simulink subsystem "Final_Project_PreAlign_20260605_152612"  (R2024a)
settings: Solver=VariableStepAuto  StartTime=0.0  StopTime=10.0  RelTol=1e-3
values from neighbouring files (symbols this model uses):
  D = hypot(Ep(:,1)-Tp(:,1)',Ep(:,2)-Tp(:,2)')    [pp_compare_stage.m]    (also in pp_diag_path.m; pp_t09_clear.m = hypot(Ep(:,1)-Tperim(:,1)', Ep(:,2)-Tperim(:,2)'); pp_tune2.m)
undefined symbols (not defined in the file or in its folder): waypoint_const
libraries: CarMaker4SL x83, simulink x2
(part 2 of 5)

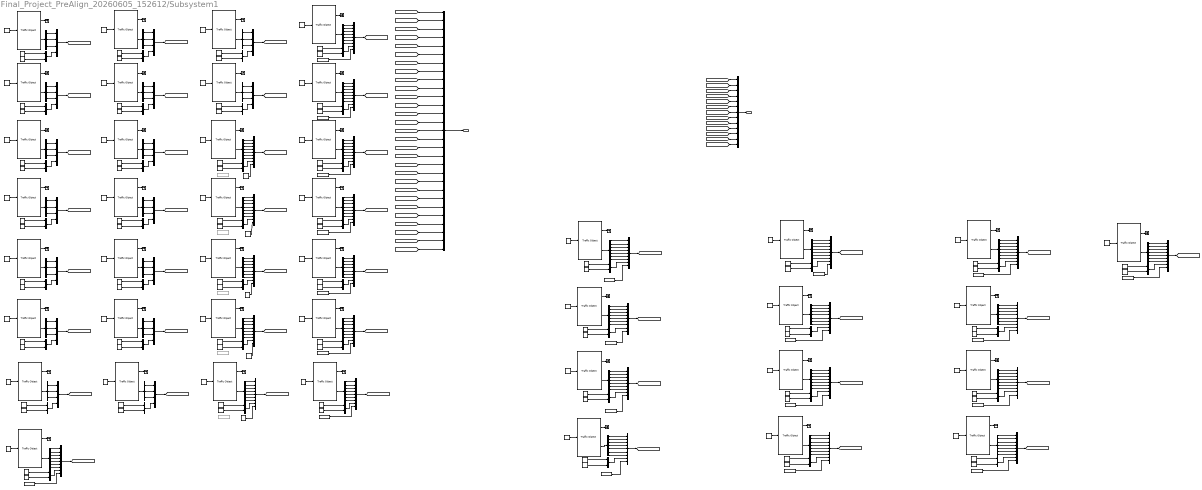
== system Final_Project_PreAlign_20260605_152612/Subsystem1 ==
  Bus Creator{,1,3..13} (13 alike) : BusCreator  Inputs=9  OutDataTypeStr=Bus: TrafficObjBus
  Bus Creator2 : BusCreator  Inputs=13  OutDataTypeStr=Bus: AllTrafficBus
  Bus Selector{,1..5,10..13,16..17,20..21,24..25} (16 alike) : BusSelector  OutputSignals=t_0 x,t_0 y,r_zyx z
  Bus Selector{6..9,14..15,18..19,22..23,26..41} (26 alike) : BusSelector  OutputSignals=t_0 x,t_0 y,r_zyx z,v_0 x,v_0 y,a_0 x,a_0 y
  Constant1 : Constant  Value=8
  Constant10 : Constant  Value=7
  Constant100 : Constant  Value=21
  Constant{7,9,12,14,16,18,20,22,30..31,34,38,42,44,47..48,51,53,59..60,63,65,71..72,75,77,83..85,89..90,95..96,101,103,108..109,113..114,119..120,125} (42 alike) : Constant  Value=4.47
  Constant102 : Constant  Value=16
  Constant{5,8,11,13,15,17,19,21,23,28,33,35,37,39,43,45,50,52,54,57,62,64,66,69,74,76,78,81,86,91..92,97..98,104..105,110..111,115..116,121..122,126} (42 alike) : Constant  Value=1.97
  Constant106 : Constant  Value=22
  Constant107 : Constant  Value=23
  Constant112 : Constant  Value=25
  Constant117 : Constant  Value=26
  Constant118 : Constant  Value=27
  Constant123 : Constant  Value=24
  Constant124 : Constant  Value=28
  Constant{36,131..135} (6 alike) : Constant  Value=0
  Constant2 : Constant  Value=9
  Constant24 : Constant  Value=22
  Constant25 : Constant  Value=23
  Constant26 : Constant  Value=2
  Constant27 : Constant
  Constant29 : Constant  Value=16
  Constant3 : Constant  Value=14
  Constant32 : Constant  Value=10
  Constant4 : Constant  Value=15
  Constant40 : Constant  Value=24
  Constant41 : Constant  Value=3
  Constant46 : Constant  Value=17
  Constant49 : Constant  Value=11
  Constant55 : Constant  Value=25
  Constant56 : Constant  Value=4
  Constant58 : Constant  Value=18
  Constant6 : Constant  Value=21
  Constant61 : Constant  Value=12
  Constant67 : Constant  Value=26
  Constant68 : Constant  Value=5
  Constant70 : Constant  Value=19
  Constant73 : Constant  Value=13
  Constant79 : Constant  Value=27
  Constant80 : Constant  Value=6
  Constant82 : Constant  Value=20
  Constant87 : Constant  Value=28
  Constant88 : Constant  Value=17
  Constant93 : Constant  Value=18
  Constant94 : Constant  Value=19
  Constant99 : Constant  Value=20
  Mux{1,4,6,8,11,14,16,18..19,21,23,26,28,30,32..33,35,38..39,41,43,46..47,49,51,54..55,57..58,60..72} (42 alike) : Mux  Inputs=2
  Mux{2..3,5,7,10,13,22,25,27,29,34,37,42,45,50,53} (16 alike) : Mux
  Mux{12,15,17,20,24,31,36,40,44,48,52,56,59} (13 alike) : Mux  Inputs=9
  Mux9 : Mux  Inputs=29
  Read CM Dict : CarMaker4SL/Read CM Dict  xname=Traffic.T27.rzv  xsync=off  xstime=Continuous
  Read CM Dict1 : CarMaker4SL/Read CM Dict  Commented=on  xname=Traffic.T16.rzv  xsync=off  xstime=Continuous
  Read CM Dict10 : CarMaker4SL/Read CM Dict  xname=Traffic.T25.rzv  xsync=off  xstime=Continuous
  Read CM Dict11 : CarMaker4SL/Read CM Dict  xname=Traffic.T26.rzv  xsync=off  xstime=Continuous
  Read CM Dict12 : CarMaker4SL/Read CM Dict  xname=Traffic.T28.rzv  xsync=off  xstime=Continuous
  Read CM Dict13 : CarMaker4SL/Read CM Dict  xname=Traffic.T17.rzv  xsync=off  xstime=Continuous
  Read CM Dict14 : CarMaker4SL/Read CM Dict  xname=Traffic.T19.rzv  xsync=off  xstime=Continuous
  Read CM Dict15 : CarMaker4SL/Read CM Dict  xname=Traffic.T18.rzv  xsync=off  xstime=Continuous
  Read CM Dict16 : CarMaker4SL/Read CM Dict  xname=Traffic.T16.rzv  xsync=off  xstime=Continuous
  Read CM Dict17 : CarMaker4SL/Read CM Dict  xname=Traffic.T21.rzv  xsync=off  xstime=Continuous
  Read CM Dict18 : CarMaker4SL/Read CM Dict  xname=Traffic.T23.rzv  xsync=off  xstime=Continuous
  Read CM Dict19 : CarMaker4SL/Read CM Dict  xname=Traffic.T22.rzv  xsync=off  xstime=Continuous
  Read CM Dict2 : CarMaker4SL/Read CM Dict  Commented=on  xname=Traffic.T17.rzv  xsync=off  xstime=Continuous
  Read CM Dict20 : CarMaker4SL/Read CM Dict  xname=Traffic.T20.rzv  xsync=off  xstime=Continuous
  Read CM Dict21 : CarMaker4SL/Read CM Dict  xname=Traffic.T25.rzv  xsync=off  xstime=Continuous
  Read CM Dict22 : CarMaker4SL/Read CM Dict  xname=Traffic.T27.rzv  xsync=off  xstime=Continuous
  Read CM Dict23 : CarMaker4SL/Read CM Dict  xname=Traffic.T26.rzv  xsync=off  xstime=Continuous
  Read CM Dict24 : CarMaker4SL/Read CM Dict  xname=Traffic.T24.rzv  xsync=off  xstime=Continuous
  Read CM Dict25 : CarMaker4SL/Read CM Dict  xname=Traffic.T28.rzv  xsync=off  xstime=Continuous
  Read CM Dict3 : CarMaker4SL/Read CM Dict  Commented=on  xname=Traffic.T18.rzv  xsync=off  xstime=Continuous
  Read CM Dict4 : CarMaker4SL/Read CM Dict  Commented=on  xname=Traffic.T19.rzv  xsync=off  xstime=Continuous
  Read CM Dict5 : CarMaker4SL/Read CM Dict  Commented=on  xname=Traffic.T20.rzv  xsync=off  xstime=Continuous
  Read CM Dict6 : CarMaker4SL/Read CM Dict  xname=Traffic.T21.rzv  xsync=off  xstime=Continuous
  Read CM Dict7 : CarMaker4SL/Read CM Dict  xname=Traffic.T22.rzv  xsync=off  xstime=Continuous
  Read CM Dict8 : CarMaker4SL/Read CM Dict  xname=Traffic.T23.rzv  xsync=off  xstime=Continuous
  Read CM Dict9 : CarMaker4SL/Read CM Dict  xname=Traffic.T24.rzv  xsync=off  xstime=Continuous
  Terminator{1..42} (42 alike) : Terminator
  Traffic Object1 : CarMaker4SL/Traffic Object  xname=T07  ximode=Traffic Id  xstime=Inherited
      settings: SourceProductName=CarMaker4SL
  Traffic Object10 : CarMaker4SL/Traffic Object  xname=T23  ximode=Traffic Id  xstime=Inherited
      settings: SourceProductName=CarMaker4SL
  Traffic Object11 : CarMaker4SL/Traffic Object  xname=T03  ximode=Traffic Id  xstime=Inherited
      settings: SourceProductName=CarMaker4SL
  Traffic Object12 : CarMaker4SL/Traffic Object  xname=T10  ximode=Traffic Id  xstime=Inherited
      settings: SourceProductName=CarMaker4SL
  Traffic Object13 : CarMaker4SL/Traffic Object  xname=T00  ximode=Traffic Id  xstime=Inherited
      settings: SourceProductName=CarMaker4SL
  Traffic Object14 : CarMaker4SL/Traffic Object  xname=T17  ximode=Traffic Id  xstime=Inherited
      settings: SourceProductName=CarMaker4SL
  Traffic Object15 : CarMaker4SL/Traffic Object  xname=T01  ximode=Traffic Id  xstime=Inherited
      settings: SourceProductName=CarMaker4SL
  Traffic Object16 : CarMaker4SL/Traffic Object  xname=T24  ximode=Traffic Id  xstime=Inherited
      settings: SourceProductName=CarMaker4SL
  Traffic Object17 : CarMaker4SL/Traffic Object  xname=T04  ximode=Traffic Id  xstime=Inherited
      settings: SourceProductName=CarMaker4SL
  Traffic Object18 : CarMaker4SL/Traffic Object  xname=T11  ximode=Traffic Id  xstime=Inherited
      settings: SourceProductName=CarMaker4SL
  Traffic Object19 : CarMaker4SL/Traffic Object  xname=T18  ximode=Traffic Id  xstime=Inherited
      settings: SourceProductName=CarMaker4SL
  Traffic Object2 : CarMaker4SL/Traffic Object  xname=T08  ximode=Traffic Id  xstime=Inherited
      settings: SourceProductName=CarMaker4SL
  Traffic Object20 : CarMaker4SL/Traffic Object  xname=T25  ximode=Traffic Id  xstime=Inherited
      settings: SourceProductName=CarMaker4SL
  Traffic Object21 : CarMaker4SL/Traffic Object  xname=T05  ximode=Traffic Id  xstime=Inherited
      settings: SourceProductName=CarMaker4SL
  Traffic Object22 : CarMaker4SL/Traffic Object  xname=T12  ximode=Traffic Id  xstime=Inherited
      settings: SourceProductName=CarMaker4SL
  Traffic Object23 : CarMaker4SL/Traffic Object  xname=T19  ximode=Traffic Id  xstime=Inherited
      settings: SourceProductName=CarMaker4SL
  Traffic Object24 : CarMaker4SL/Traffic Object  xname=T26  ximode=Traffic Id  xstime=Inherited
      settings: SourceProductName=CarMaker4SL
  Traffic Object25 : CarMaker4SL/Traffic Object  xname=T06  ximode=Traffic Id  xstime=Inherited
      settings: SourceProductName=CarMaker4SL
  Traffic Object26 : CarMaker4SL/Traffic Object  xname=T13  ximode=Traffic Id  xstime=Inherited
      settings: SourceProductName=CarMaker4SL
  Traffic Object27 : CarMaker4SL/Traffic Object  xname=T20  ximode=Traffic Id  xstime=Inherited
      settings: SourceProductName=CarMaker4SL
  Traffic Object28 : CarMaker4SL/Traffic Object  xname=T27  ximode=Traffic Id  xstime=Inherited
      settings: SourceProductName=CarMaker4SL
  Traffic Object29 : CarMaker4SL/Traffic Object  xname=T28  ximode=Traffic Id  xstime=Inherited
      settings: SourceProductName=CarMaker4SL
  Traffic Object3 : CarMaker4SL/Traffic Object  xname=T02  ximode=Traffic Id  xstime=Inherited
      settings: SourceProductName=CarMaker4SL
  Traffic Object30 : CarMaker4SL/Traffic Object  xname=T17  ximode=Traffic Id  xstime=Inherited
      settings: SourceProductName=CarMaker4SL
  Traffic Object31 : CarMaker4SL/Traffic Object  xname=T19  ximode=Traffic Id  xstime=Inherited
      settings: SourceProductName=CarMaker4SL
  Traffic Object32 : CarMaker4SL/Traffic Object  xname=T18  ximode=Traffic Id  xstime=Inherited
      settings: SourceProductName=CarMaker4SL
  Traffic Object33 : CarMaker4SL/Traffic Object  xname=T21  ximode=Traffic Id  xstime=Inherited
      settings: SourceProductName=CarMaker4SL
  Traffic Object34 : CarMaker4SL/Traffic Object  xname=T23  ximode=Traffic Id  xstime=Inherited
      settings: SourceProductName=CarMaker4SL
  Traffic Object35 : CarMaker4SL/Traffic Object  xname=T16  ximode=Traffic Id  xstime=Inherited
      settings: SourceProductName=CarMaker4SL
  Traffic Object36 : CarMaker4SL/Traffic Object  xname=T22  ximode=Traffic Id  xstime=Inherited
      settings: SourceProductName=CarMaker4SL
  Traffic Object37 : CarMaker4SL/Traffic Object  xname=T20  ximode=Traffic Id  xstime=Inherited
      settings: SourceProductName=CarMaker4SL
  Traffic Object38 : CarMaker4SL/Traffic Object  xname=T25  ximode=Traffic Id  xstime=Inherited
      settings: SourceProductName=CarMaker4SL
  Traffic Object39 : CarMaker4SL/Traffic Object  xname=T27  ximode=Traffic Id  xstime=Inherited
      settings: SourceProductName=CarMaker4SL
  Traffic Object4 : CarMaker4SL/Traffic Object  xname=T14  ximode=Traffic Id  xstime=Inherited
      settings: SourceProductName=CarMaker4SL
  Traffic Object40 : CarMaker4SL/Traffic Object  xname=T26  ximode=Traffic Id  xstime=Inherited
      settings: SourceProductName=CarMaker4SL
  Traffic Object41 : CarMaker4SL/Traffic Object  xname=T24  ximode=Traffic Id  xstime=Inherited
      settings: SourceProductName=CarMaker4SL
  Traffic Object42 : CarMaker4SL/Traffic Object  xname=T28  ximode=Traffic Id  xstime=Inherited
      settings: SourceProductName=CarMaker4SL
  Traffic Object5 : CarMaker4SL/Traffic Object  xname=T15  ximode=Traffic Id  xstime=Inherited
      settings: SourceProductName=CarMaker4SL
  Traffic Object6 : CarMaker4SL/Traffic Object  xname=T09  ximode=Traffic Id  xstime=Inherited
      settings: SourceProductName=CarMaker4SL
  Traffic Object7 : CarMaker4SL/Traffic Object  xname=T21  ximode=Traffic Id  xstime=Inherited
      settings: SourceProductName=CarMaker4SL
  Traffic Object8 : CarMaker4SL/Traffic Object  xname=T22  ximode=Traffic Id  xstime=Inherited
      settings: SourceProductName=CarMaker4SL
  Traffic Object9 : CarMaker4SL/Traffic Object  xname=T16  ximode=Traffic Id  xstime=Inherited
      settings: SourceProductName=CarMaker4SL
  Traffic_Info : Outport
  Outport : Outport  Port=2
  wires:
  Constant135/1 -> Mux56/9
  Constant134/1 -> Mux48/9
  Constant133/1 -> Mux40/9
  Constant132/1 -> Mux31/9
  Constant131/1 -> Mux20/9
  Read CM Dict16/1 -> Bus Creator/9
  Read CM Dict13/1 -> Bus Creator3/9
  Read CM Dict15/1 -> Bus Creator1/9
  Read CM Dict14/1 -> Bus Creator4/9
  Read CM Dict20/1 -> Bus Creator5/9
  [Traffic_Info_16_Bus] -> Bus Creator2/1  "t16"
  [Traffic_Info_17_Bus] -> Bus Creator2/2  "t17"
  [Traffic_Info_18_Bus] -> Bus Creator2/3  "t18"
  [Traffic_Info_19_Bus] -> Bus Creator2/4  "t19"
  [Traffic_Info_20_Bus] -> Bus Creator2/5  "t20"
  [Traffic_Info_21_Bus] -> Bus Creator2/6  "t21"
  [Traffic_Info_22_Bus] -> Bus Creator2/7  "t22"
  [Traffic_Info_23_Bus] -> Bus Creator2/8  "t23"
  [Traffic_Info_24_Bus] -> Bus Creator2/9  "t24"
  [Traffic_Info_25_Bus] -> Bus Creator2/10  "t25"
  [Traffic_Info_26_Bus] -> Bus Creator2/11  "t26"
  [Traffic_Info_27_Bus] -> Bus Creator2/12  "t27"
  [Traffic_Info_28_Bus] -> Bus Creator2/13  "t28"
  Bus Selector41/7 -> Bus Creator13/7  "<a_0 y>"
  Bus Selector41/1 -> Bus Creator13/1  "<t_0 x>"
  Constant125/1 -> Mux72/1
  Bus Selector41/2 -> Bus Creator13/2  "<t_0 y>"
  Traffic Object42/1 -> Terminator42/1
  Bus Selector41/6 -> Bus Creator13/6  "<a_0 x>"
  Traffic Object42/2 -> Bus Selector41/1
  Bus Creator13/1 -> [Traffic_Info_28_Bus]
  Mux72/1 -> Bus Creator13/8  "Traffic_Boundary"
  Bus Selector41/4 -> Bus Creator13/4  "<v_0 x>"
  Constant126/1 -> Mux72/2
  Bus Selector41/5 -> Bus Creator13/5  "<v_0 y>"
  Bus Selector41/3 -> Bus Creator13/3  "<r_zyx z>"
  Read CM Dict25/1 -> Bus Creator13/9  "Yawrate"
  Constant124/1 -> Traffic Object42/1
  Constant114/1 -> Mux70/1
  Bus Selector39/3 -> Bus Creator10/3  "<r_zyx z>"
  Constant116/1 -> Mux68/2
  Bus Creator12/1 -> [Traffic_Info_27_Bus]
  Mux71/1 -> Bus Creator10/8  "Traffic_Boundary"
  Bus Selector39/7 -> Bus Creator10/7  "<a_0 y>"
  Traffic Object39/1 -> Terminator39/1
  Traffic Object41/2 -> Bus Selector40/1
  Bus Selector38/2 -> Bus Creator12/2  "<t_0 y>"
  Mux68/1 -> Bus Creator11/8  "Traffic_Boundary"
  Bus Selector40/6 -> Bus Creator9/6  "<a_0 x>"
  Traffic Object39/2 -> Bus Selector38/1
  Bus Selector37/5 -> Bus Creator11/5  "<v_0 y>"
  Bus Selector37/7 -> Bus Creator11/7  "<a_0 y>"
  Bus Selector40/4 -> Bus Creator9/4  "<v_0 x>"
  Traffic Object38/2 -> Bus Selector37/1
  Bus Selector39/2 -> Bus Creator10/2  "<t_0 y>"
  Constant112/1 -> Traffic Object38/1
  Bus Selector40/3 -> Bus Creator9/3  "<r_zyx z>"
  Constant119/1 -> Mux69/1
  Bus Selector40/5 -> Bus Creator9/5  "<v_0 y>"
  Traffic Object40/2 -> Bus Selector39/1
  Bus Selector38/1 -> Bus Creator12/1  "<t_0 x>"
  Constant120/1 -> Mux71/1
  Bus Selector38/7 -> Bus Creator12/7  "<a_0 y>"
  Bus Selector40/2 -> Bus Creator9/2  "<t_0 y>"
  Traffic Object40/1 -> Terminator40/1
  Constant117/1 -> Traffic Object40/1
  Bus Selector40/1 -> Bus Creator9/1  "<t_0 x>"
  Read CM Dict23/1 -> Bus Creator10/9  "Yawrate"
  Constant115/1 -> Mux70/2
  Bus Selector39/1 -> Bus Creator10/1  "<t_0 x>"
  Bus Selector39/6 -> Bus Creator10/6  "<a_0 x>"
  Constant121/1 -> Mux71/2
  Constant118/1 -> Traffic Object39/1
  Bus Selector37/4 -> Bus Creator11/4  "<v_0 x>"
  Constant113/1 -> Mux68/1
  Read CM Dict24/1 -> Bus Creator9/9  "Yawrate"
  Bus Selector40/7 -> Bus Creator9/7  "<a_0 y>"
  Bus Selector37/3 -> Bus Creator11/3  "<r_zyx z>"
  Bus Selector39/5 -> Bus Creator10/5  "<v_0 y>"
  Read CM Dict22/1 -> Bus Creator12/9  "Yawrate"
  Bus Selector37/2 -> Bus Creator11/2  "<t_0 y>"
  Bus Creator11/1 -> [Traffic_Info_25_Bus]
  Read CM Dict21/1 -> Bus Creator11/9  "Yawrate"
  Mux70/1 -> Bus Creator9/8  "Traffic_Boundary"
  Bus Selector37/6 -> Bus Creator11/6  "<a_0 x>"
  Bus Selector38/3 -> Bus Creator12/3  "<r_zyx z>"
  Bus Selector37/1 -> Bus Creator11/1  "<t_0 x>"
  Bus Creator9/1 -> [Traffic_Info_24_Bus]
  Traffic Object38/1 -> Terminator38/1
  Constant122/1 -> Mux69/2
  Bus Selector38/6 -> Bus Creator12/6  "<a_0 x>"
  Bus Creator10/1 -> [Traffic_Info_26_Bus]
  Bus Selector38/4 -> Bus Creator12/4  "<v_0 x>"
  Bus Selector38/5 -> Bus Creator12/5  "<v_0 y>"
  Constant123/1 -> Traffic Object41/1
  Traffic Object41/1 -> Terminator41/1
  Bus Selector39/4 -> Bus Creator10/4  "<v_0 x>"
  Mux69/1 -> Bus Creator12/8  "Traffic_Boundary"
  Constant105/1 -> Mux64/2
  Mux65/1 -> Bus Creator8/8  "Traffic_Boundary"
  Bus Selector34/1 -> Bus Creator8/1  "<t_0 x>"
  Traffic Object36/2 -> Bus Selector35/1
  Read CM Dict19/1 -> Bus Creator6/9  "Yawrate"
  Bus Selector32/1 -> Bus Creator7/1  "<t_0 x>"
  Bus Creator6/1 -> [Traffic_Info_22_Bus]
  Bus Selector34/4 -> Bus Creator8/4  "<v_0 x>"
  Bus Creator8/1 -> [Traffic_Info_23_Bus]
  Bus Selector35/4 -> Bus Creator6/4  "<v_0 x>"
  Traffic Object37/1 -> Terminator37/1
  Constant111/1 -> Mux65/2
  Constant99/1 -> Traffic Object37/1
  Bus Selector34/6 -> Bus Creator8/6  "<a_0 x>"
  Bus Selector34/5 -> Bus Creator8/5  "<v_0 y>"
  Mux64/1 -> Bus Creator7/8  "Traffic_Boundary"
  Bus Creator7/1 -> [Traffic_Info_21_Bus]
  Bus Selector34/3 -> Bus Creator8/3  "<r_zyx z>"
  Bus Selector32/2 -> Bus Creator7/2  "<t_0 y>"
  Bus Creator5/1 -> [Traffic_Info_20_Bus]
  Read CM Dict18/1 -> Bus Creator8/9  "Yawrate"
  Traffic Object33/1 -> Terminator33/1
  Bus Selector32/6 -> Bus Creator7/6  "<a_0 x>"
  Mux66/1 -> Bus Creator5/8  "Traffic_Boundary"
  Read CM Dict17/1 -> Bus Creator7/9  "Yawrate"
  Bus Selector32/4 -> Bus Creator7/4  "<v_0 x>"
  Bus Selector35/6 -> Bus Creator6/6  "<a_0 x>"
  Bus Selector32/3 -> Bus Creator7/3  "<r_zyx z>"
  Constant101/1 -> Mux64/1
  Bus Selector36/7 -> Bus Creator5/7  "<a_0 y>"
  Constant106/1 -> Traffic Object36/1
  Bus Selector32/7 -> Bus Creator7/7  "<a_0 y>"
  Constant110/1 -> Mux67/2
  Bus Selector35/5 -> Bus Creator6/5  "<v_0 y>"
  Constant107/1 -> Traffic Object34/1
  Bus Selector34/7 -> Bus Creator8/7  "<a_0 y>"
  Constant108/1 -> Mux65/1
  Bus Selector35/1 -> Bus Creator6/1  "<t_0 x>"
  Bus Selector36/2 -> Bus Creator5/2  "<t_0 y>"
  Bus Selector35/7 -> Bus Creator6/7  "<a_0 y>"
  Traffic Object36/1 -> Terminator36/1
  Constant109/1 -> Mux67/1
  Bus Selector36/1 -> Bus Creator5/1  "<t_0 x>"
  Bus Selector36/5 -> Bus Creator5/5  "<v_0 y>"
  Constant104/1 -> Mux66/2
  Constant103/1 -> Mux66/1
  Traffic Object37/2 -> Bus Selector36/1
  Bus Selector36/6 -> Bus Creator5/6  "<a_0 x>"
  Bus Selector36/3 -> Bus Creator5/3  "<r_zyx z>"
  Bus Selector36/4 -> Bus Creator5/4  "<v_0 x>"
  Traffic Object33/2 -> Bus Selector32/1
  Constant100/1 -> Traffic Object33/1
  Bus Selector32/5 -> Bus Creator7/5  "<v_0 y>"
  Bus Selector35/2 -> Bus Creator6/2  "<t_0 y>"
  Traffic Object34/2 -> Bus Selector34/1
  Bus Selector35/3 -> Bus Creator6/3  "<r_zyx z>"
  Bus Selector34/2 -> Bus Creator8/2  "<t_0 y>"
  Traffic Object34/1 -> Terminator34/1
  Mux67/1 -> Bus Creator6/8  "Traffic_Boundary"
  Bus Selector30/6 -> Bus Creator4/6  "<a_0 x>"
  Bus Creator4/1 -> [Traffic_Info_19_Bus]
  Constant98/1 -> Mux61/2
  Bus Selector30/1 -> Bus Creator4/1  "<t_0 x>"
  Mux61/1 -> Bus Creator4/8  "Traffic_Boundary"
  Bus Creator1/1 -> [Traffic_Info_18_Bus]
  Bus Selector30/2 -> Bus Creator4/2  "<t_0 y>"
  Traffic Object31/1 -> Terminator31/1
  Mux63/1 -> Bus Creator1/8  "Traffic_Boundary"
  Bus Selector30/4 -> Bus Creator4/4  "<v_0 x>"
  Bus Selector30/3 -> Bus Creator4/3  "<r_zyx z>"
  Constant95/1 -> Mux61/1
  Bus Selector31/7 -> Bus Creator1/7  "<a_0 y>"
  Bus Selector31/1 -> Bus Creator1/1  "<t_0 x>"
  Bus Selector31/5 -> Bus Creator1/5  "<v_0 y>"
  Bus Selector30/7 -> Bus Creator4/7  "<a_0 y>"
  Constant97/1 -> Mux63/2
  Constant93/1 -> Traffic Object32/1
  Constant96/1 -> Mux63/1
  Traffic Object32/2 -> Bus Selector31/1
  Traffic Object32/1 -> Terminator32/1
  Bus Selector31/6 -> Bus Creator1/6  "<a_0 x>"
  Bus Selector31/3 -> Bus Creator1/3  "<r_zyx z>"
  Bus Selector31/4 -> Bus Creator1/4  "<v_0 x>"
  Traffic Object31/2 -> Bus Selector30/1
  Constant94/1 -> Traffic Object31/1
  Bus Selector30/5 -> Bus Creator4/5  "<v_0 y>"
  Bus Selector31/2 -> Bus Creator1/2  "<t_0 y>"
  Bus Creator3/1 -> [Traffic_Info_17_Bus]
  Bus Selector29/1 -> Bus Creator3/1  "<t_0 x>"
  Mux60/1 -> Bus Creator3/8  "Traffic_Boundary"
  Bus Selector29/7 -> Bus Creator3/7  "<a_0 y>"
  Bus Selector29/5 -> Bus Creator3/5  "<v_0 y>"
  Constant89/1 -> Mux60/1
  Constant92/1 -> Mux60/2
  Constant88/1 -> Traffic Object30/1
  Traffic Object30/2 -> Bus Selector29/1
  Traffic Object30/1 -> Terminator30/1
  Bus Selector29/6 -> Bus Creator3/6  "<a_0 x>"
  Bus Selector29/3 -> Bus Creator3/3  "<r_zyx z>"
  Bus Selector29/4 -> Bus Creator3/4  "<v_0 x>"
  Bus Selector29/2 -> Bus Creator3/2  "<t_0 y>"
  Bus Creator2/1 -> Outport/1
  Bus Creator/1 -> [Traffic_Info_16_Bus]
  Constant91/1 -> Mux62/2
  Bus Selector33/5 -> Bus Creator/5  "<v_0 y>"
  Bus Selector33/4 -> Bus Creator/4  "<v_0 x>"
  Bus Selector33/3 -> Bus Creator/3  "<r_zyx z>"
  Bus Selector33/7 -> Bus Creator/7  "<a_0 y>"
  Bus Selector33/6 -> Bus Creator/6  "<a_0 x>"
  Mux62/1 -> Bus Creator/8  "Traffic_Boundary"
  Traffic Object35/2 -> Bus Selector33/1
  Bus Selector33/2 -> Bus Creator/2  "<t_0 y>"
  Traffic Object35/1 -> Terminator35/1
  Bus Selector33/1 -> Bus Creator/1  "<t_0 x>"
  Constant90/1 -> Mux62/1
  Constant102/1 -> Traffic Object35/1
  Mux9/1 -> Traffic_Info/1
  Traffic Object29/1 -> Terminator29/1
  Bus Selector28/1 -> Mux59/1  "<t_0 x>"
  Bus Selector28/2 -> Mux59/2  "<t_0 y>"
  Bus Selector28/4 -> Mux59/4  "<v_0 x>"
  Constant87/1 -> Traffic Object29/1
  Traffic Object29/2 -> Bus Selector28/1
  Constant86/1 -> Mux58/2
  Mux59/1 -> [Traffic_Info_28]
  Constant85/1 -> Mux58/1
  Bus Selector28/3 -> Mux59/3  "<r_zyx z>"
  Bus Selector28/6 -> Mux59/6  "<a_0 x>"
  Bus Selector28/7 -> Mux59/7  "<a_0 y>"
  Bus Selector28/5 -> Mux59/5  "<v_0 y>"
  Read CM Dict12/1 -> Mux59/9  "Yawrate"
  Mux58/1 -> Mux59/8  "Traffic_Boundary"
  Traffic Object24/1 -> Terminator24/1
  Bus Selector23/1 -> Mux44/1  "<t_0 x>"
  Bus Selector23/2 -> Mux44/2  "<t_0 y>"
  Bus Selector23/4 -> Mux44/4  "<v_0 x>"
  Constant67/1 -> Traffic Object24/1
  Traffic Object24/2 -> Bus Selector23/1
  Constant66/1 -> Mux43/2
  Mux44/1 -> [Traffic_Info_26]
  Constant65/1 -> Mux43/1
  Bus Selector23/3 -> Mux44/3  "<r_zyx z>"
  Bus Selector23/6 -> Mux44/6  "<a_0 x>"
  Bus Selector23/7 -> Mux44/7  "<a_0 y>"
  Bus Selector23/5 -> Mux44/5  "<v_0 y>"
  Read CM Dict11/1 -> Mux44/9  "Yawrate"
  Mux43/1 -> Mux44/8  "Traffic_Boundary"
  Traffic Object20/1 -> Terminator20/1
  Bus Selector19/1 -> Mux36/1  "<t_0 x>"
  Bus Selector19/2 -> Mux36/2  "<t_0 y>"
  Bus Selector19/4 -> Mux36/4  "<v_0 x>"
  Constant55/1 -> Traffic Object20/1
  Traffic Object20/2 -> Bus Selector19/1
  Constant54/1 -> Mux35/2
  Mux36/1 -> [Traffic_Info_25]
  Constant53/1 -> Mux35/1
  Bus Selector19/3 -> Mux36/3  "<r_zyx z>"
  Bus Selector19/6 -> Mux36/6  "<a_0 x>"
  Bus Selector19/7 -> Mux36/7  "<a_0 y>"
  Bus Selector19/5 -> Mux36/5  "<v_0 y>"
  Read CM Dict10/1 -> Mux36/9  "Yawrate"
  Mux35/1 -> Mux36/8  "Traffic_Boundary"
  Traffic Object16/1 -> Terminator16/1
  Bus Selector15/1 -> Mux24/1  "<t_0 x>"
  Bus Selector15/2 -> Mux24/2  "<t_0 y>"
  Bus Selector15/4 -> Mux24/4  "<v_0 x>"
  Constant40/1 -> Traffic Object16/1
  Traffic Object16/2 -> Bus Selector15/1
  Constant39/1 -> Mux23/2
  Mux24/1 -> [Traffic_Info_24]
  Constant38/1 -> Mux23/1
  Bus Selector15/3 -> Mux24/3  "<r_zyx z>"
  Bus Selector15/6 -> Mux24/6  "<a_0 x>"
  Bus Selector15/7 -> Mux24/7  "<a_0 y>"
  Bus Selector15/5 -> Mux24/5  "<v_0 y>"
  Read CM Dict9/1 -> Mux24/9  "Yawrate"
  Mux23/1 -> Mux24/8  "Traffic_Boundary"
  Traffic Object10/1 -> Terminator10/1
  Bus Selector9/1 -> Mux12/1  "<t_0 x>"
  Bus Selector9/2 -> Mux12/2  "<t_0 y>"
  Bus Selector9/4 -> Mux12/4  "<v_0 x>"
  Constant25/1 -> Traffic Object10/1
  Traffic Object10/2 -> Bus Selector9/1
  Constant19/1 -> Mux11/2
  Mux12/1 -> [Traffic_Info_23]
  Constant18/1 -> Mux11/1
  Bus Selector9/3 -> Mux12/3  "<r_zyx z>"
  Bus Selector9/6 -> Mux12/6  "<a_0 x>"
  Bus Selector9/7 -> Mux12/7  "<a_0 y>"
  Bus Selector9/5 -> Mux12/5  "<v_0 y>"
  Read CM Dict8/1 -> Mux12/9  "Yawrate"
  Mux11/1 -> Mux12/8  "Traffic_Boundary"
  Traffic Object8/1 -> Terminator8/1
  Bus Selector7/1 -> Mux17/1  "<t_0 x>"
  Bus Selector7/2 -> Mux17/2  "<t_0 y>"
  Bus Selector7/4 -> Mux17/4  "<v_0 x>"
  Constant24/1 -> Traffic Object8/1
  Traffic Object8/2 -> Bus Selector7/1
  Constant23/1 -> Mux16/2
  Mux17/1 -> [Traffic_Info_22]
  Constant22/1 -> Mux16/1
  Bus Selector7/3 -> Mux17/3  "<r_zyx z>"
  Bus Selector7/6 -> Mux17/6  "<a_0 x>"
  Bus Selector7/7 -> Mux17/7  "<a_0 y>"
  Bus Selector7/5 -> Mux17/5  "<v_0 y>"
  Read CM Dict7/1 -> Mux17/9  "Yawrate"
  Mux16/1 -> Mux17/8  "Traffic_Boundary"
  Traffic Object7/1 -> Terminator7/1
  Bus Selector6/1 -> Mux15/1  "<t_0 x>"
  Bus Selector6/2 -> Mux15/2  "<t_0 y>"
  Bus Selector6/4 -> Mux15/4  "<v_0 x>"
  Constant6/1 -> Traffic Object7/1
  Traffic Object7/2 -> Bus Selector6/1
  Constant21/1 -> Mux14/2
  Mux15/1 -> [Traffic_Info_21]
  Constant20/1 -> Mux14/1
  Bus Selector6/3 -> Mux15/3  "<r_zyx z>"
  Bus Selector6/6 -> Mux15/6  "<a_0 x>"
  Bus Selector6/7 -> Mux15/7  "<a_0 y>"
  Bus Selector6/5 -> Mux15/5  "<v_0 y>"
  Read CM Dict6/1 -> Mux15/9  "Yawrate"
  Mux14/1 -> Mux15/8  "Traffic_Boundary"
  Traffic Object27/1 -> Terminator27/1
  Bus Selector26/1 -> Mux56/1  "<t_0 x>"
  Bus Selector26/2 -> Mux56/2  "<t_0 y>"
  Bus Selector26/4 -> Mux56/4  "<v_0 x>"
  Constant82/1 -> Traffic Object27/1
  Traffic Object27/2 -> Bus Selector26/1
  Constant76/1 -> Mux55/2
  Mux56/1 -> [Traffic_Info_20]
  Constant75/1 -> Mux55/1
  Bus Selector26/3 -> Mux56/3  "<r_zyx z>"
  Bus Selector26/6 -> Mux56/6  "<a_0 x>"
  Bus Selector26/7 -> Mux56/7  "<a_0 y>"
  Bus Selector26/5 -> Mux56/5  "<v_0 y>"
  Mux55/1 -> Mux56/8  "Traffic_Boundary"
  Traffic Object23/1 -> Terminator23/1
  Bus Selector22/1 -> Mux48/1  "<t_0 x>"
  Bus Selector22/2 -> Mux48/2  "<t_0 y>"
  Bus Selector22/4 -> Mux48/4  "<v_0 x>"
  Constant70/1 -> Traffic Object23/1
  Traffic Object23/2 -> Bus Selector22/1
  Constant64/1 -> Mux47/2
  Mux48/1 -> [Traffic_Info_19]
  Constant63/1 -> Mux47/1
  Bus Selector22/3 -> Mux48/3  "<r_zyx z>"
  Bus Selector22/6 -> Mux48/6  "<a_0 x>"
  Bus Selector22/7 -> Mux48/7  "<a_0 y>"
  Bus Selector22/5 -> Mux48/5  "<v_0 y>"
  Mux47/1 -> Mux48/8  "Traffic_Boundary"
  Traffic Object19/1 -> Terminator19/1
  Bus Selector18/1 -> Mux40/1  "<t_0 x>"
  Bus Selector18/2 -> Mux40/2  "<t_0 y>"
  Bus Selector18/4 -> Mux40/4  "<v_0 x>"
  Constant58/1 -> Traffic Object19/1
  Traffic Object19/2 -> Bus Selector18/1
  Constant52/1 -> Mux39/2
  Mux40/1 -> [Traffic_Info_18]
  Constant51/1 -> Mux39/1
  Bus Selector18/3 -> Mux40/3  "<r_zyx z>"
  Bus Selector18/6 -> Mux40/6  "<a_0 x>"
  Bus Selector18/7 -> Mux40/7  "<a_0 y>"
  Bus Selector18/5 -> Mux40/5  "<v_0 y>"
  Mux39/1 -> Mux40/8  "Traffic_Boundary"
  Traffic Object14/1 -> Terminator14/1
  Bus Selector14/1 -> Mux31/1  "<t_0 x>"
  Bus Selector14/2 -> Mux31/2  "<t_0 y>"
  Bus Selector14/4 -> Mux31/4  "<v_0 x>"
  Constant46/1 -> Traffic Object14/1
  Traffic Object14/2 -> Bus Selector14/1
  Constant35/1 -> Mux30/2
  Mux31/1 -> [Traffic_Info_17]
  Constant34/1 -> Mux30/1
  Bus Selector14/3 -> Mux31/3  "<r_zyx z>"
  Bus Selector14/6 -> Mux31/6  "<a_0 x>"
  Bus Selector14/7 -> Mux31/7  "<a_0 y>"
  Bus Selector14/5 -> Mux31/5  "<v_0 y>"
  Mux30/1 -> Mux31/8  "Traffic_Boundary"
  Traffic Object9/1 -> Terminator9/1
  Bus Selector8/1 -> Mux20/1  "<t_0 x>"
  Bus Selector8/2 -> Mux20/2  "<t_0 y>"
  Bus Selector8/4 -> Mux20/4  "<v_0 x>"
  Constant29/1 -> Traffic Object9/1
  Traffic Object9/2 -> Bus Selector8/1
  Constant13/1 -> Mux19/2
  Mux20/1 -> [Traffic_Info_16]
  Constant12/1 -> Mux19/1
  Bus Selector8/3 -> Mux20/3  "<r_zyx z>"
  Bus Selector8/6 -> Mux20/6  "<a_0 x>"
  Bus Selector8/7 -> Mux20/7  "<a_0 y>"
  Bus Selector8/5 -> Mux20/5  "<v_0 y>"
  Mux19/1 -> Mux20/8  "Traffic_Boundary"
  Read CM Dict/1 -> Mux52/9  "Yawrate"
  Mux51/1 -> Mux52/8  "Traffic_Boundary"
  Bus Selector27/7 -> Mux52/7  "<a_0 y>"
  Bus Selector27/6 -> Mux52/6  "<a_0 x>"
  Bus Selector27/5 -> Mux52/5  "<v_0 y>"
  Bus Selector27/4 -> Mux52/4  "<v_0 x>"
  [Traffic_Info_28] -> Mux9/29  "T28"
  Constant10/1 -> Traffic Object1/1
  Traffic Object1/1 -> Terminator1/1
  Traffic Object2/1 -> Terminator2/1
  Constant1/1 -> Traffic Object2/1
  Traffic Object4/1 -> Terminator4/1
  Constant3/1 -> Traffic Object4/1
  Constant4/1 -> Traffic Object5/1
  Traffic Object5/1 -> Terminator5/1
  Traffic Object1/2 -> Bus Selector/1
  Bus Selector/1 -> Mux2/1  "<t_0 x>"
  Bus Selector/2 -> Mux2/2  "<t_0 y>"
  Bus Selector/3 -> Mux2/3  "<r_zyx z>"
  Bus Selector1/2 -> Mux10/2  "<t_0 y>"
  Mux10/1 -> [Traffic_Info_08]
  Bus Selector1/1 -> Mux10/1  "<t_0 x>"
  Bus Selector1/3 -> Mux10/3  "<r_zyx z>"
  Traffic Object2/2 -> Bus Selector1/1
  Bus Selector3/2 -> Mux5/2  "<t_0 y>"
  Mux5/1 -> [Traffic_Info_14]
  Bus Selector3/1 -> Mux5/1  "<t_0 x>"
  Bus Selector3/3 -> Mux5/3  "<r_zyx z>"
  Traffic Object4/2 -> Bus Selector3/1
  Bus Selector4/2 -> Mux7/2  "<t_0 y>"
  Mux7/1 -> [Traffic_Info_15]
  Bus Selector4/1 -> Mux7/1  "<t_0 x>"
  Bus Selector4/3 -> Mux7/3  "<r_zyx z>"
  Traffic Object5/2 -> Bus Selector4/1
  Mux2/1 -> [Traffic_Info_07]
  [Traffic_Info_00] -> Mux9/1  "T00"
  [Traffic_Info_01] -> Mux9/2  "T01"
  [Traffic_Info_02] -> Mux9/3  "T02"
  [Traffic_Info_06] -> Mux9/7  "T06"
  [Traffic_Info_05] -> Mux9/6  "T05"
  [Traffic_Info_04] -> Mux9/5  "T04"
  [Traffic_Info_03] -> Mux9/4  "T03"
  Constant8/1 -> Mux1/2
  Mux1/1 -> Mux2/4
  Constant7/1 -> Mux1/1
  Constant11/1 -> Mux8/2
  Constant9/1 -> Mux8/1
  Mux8/1 -> Mux10/4
  Constant15/1 -> Mux4/2
  Constant14/1 -> Mux4/1
  Mux4/1 -> Mux5/4
  Constant17/1 -> Mux6/2
  Constant16/1 -> Mux6/1
  Mux6/1 -> Mux7/4
  Constant37/1 -> Mux33/2
  Traffic Object13/2 -> Bus Selector12/1
  Mux26/1 -> Mux29/4
  Bus Selector12/1 -> Mux29/1  "<t_0 x>"
  Constant36/1 -> Traffic Object13/1
  Constant42/1 -> Mux26/1
  Mux27/1 -> [Traffic_Info_01]
  Traffic Object15/2 -> Bus Selector13/1
  Traffic Object13/1 -> Terminator13/1
  Traffic Object15/1 -> Terminator15/1
  Bus Selector12/2 -> Mux29/2  "<t_0 y>"
  Constant44/1 -> Mux33/1
  Bus Selector13/1 -> Mux27/1  "<t_0 x>"
  Mux33/1 -> Mux27/4
  Bus Selector13/3 -> Mux27/3  "<r_zyx z>"
  Bus Selector13/2 -> Mux27/2  "<t_0 y>"
  Constant43/1 -> Mux26/2
  Mux29/1 -> [Traffic_Info_00]
  Bus Selector12/3 -> Mux29/3  "<r_zyx z>"
  Constant27/1 -> Traffic Object15/1
  Constant5/1 -> Mux21/2
  Constant26/1 -> Traffic Object3/1
  Bus Selector5/2 -> Mux13/2  "<t_0 y>"
  Mux3/1 -> [Traffic_Info_09]
  Bus Selector2/2 -> Mux3/2  "<t_0 y>"
  Mux21/1 -> Mux3/4
  Traffic Object6/2 -> Bus Selector2/1
  Bus Selector2/1 -> Mux3/1  "<t_0 x>"
  Traffic Object6/1 -> Terminator6/1
  Bus Selector2/3 -> Mux3/3  "<r_zyx z>"
  Constant28/1 -> Mux18/2
  Traffic Object3/2 -> Bus Selector5/1
  Traffic Object3/1 -> Terminator3/1
  Mux13/1 -> [Traffic_Info_02]
  Bus Selector5/3 -> Mux13/3  "<r_zyx z>"
  Constant2/1 -> Traffic Object6/1
  Bus Selector5/1 -> Mux13/1  "<t_0 x>"
  Mux18/1 -> Mux13/4
  Constant30/1 -> Mux18/1
  Constant31/1 -> Mux21/1
  Constant33/1 -> Mux32/2
  Constant41/1 -> Traffic Object11/1
  Bus Selector11/2 -> Mux25/2  "<t_0 y>"
  Mux22/1 -> [Traffic_Info_10]
  Bus Selector10/2 -> Mux22/2  "<t_0 y>"
  Mux32/1 -> Mux22/4
  Traffic Object12/2 -> Bus Selector10/1
  Bus Selector10/1 -> Mux22/1  "<t_0 x>"
  Traffic Object12/1 -> Terminator12/1
  Bus Selector10/3 -> Mux22/3  "<r_zyx z>"
  Constant45/1 -> Mux28/2
  Traffic Object11/2 -> Bus Selector11/1
  Traffic Object11/1 -> Terminator11/1
  Mux25/1 -> [Traffic_Info_03]
  Bus Selector11/3 -> Mux25/3  "<r_zyx z>"
  Constant32/1 -> Traffic Object12/1
  Bus Selector11/1 -> Mux25/1  "<t_0 x>"
  Mux28/1 -> Mux25/4
  Constant47/1 -> Mux28/1
  Constant48/1 -> Mux32/1
  Constant50/1 -> Mux41/2
  Constant56/1 -> Traffic Object17/1
  Bus Selector17/2 -> Mux37/2  "<t_0 y>"
  Mux34/1 -> [Traffic_Info_11]
  Bus Selector16/2 -> Mux34/2  "<t_0 y>"
  Mux41/1 -> Mux34/4
  Traffic Object18/2 -> Bus Selector16/1
  Bus Selector16/1 -> Mux34/1  "<t_0 x>"
  Traffic Object18/1 -> Terminator18/1
  Bus Selector16/3 -> Mux34/3  "<r_zyx z>"
  Constant57/1 -> Mux38/2
  Traffic Object17/2 -> Bus Selector17/1
  Traffic Object17/1 -> Terminator17/1
  Mux37/1 -> [Traffic_Info_04]
  Bus Selector17/3 -> Mux37/3  "<r_zyx z>"
  Constant49/1 -> Traffic Object18/1
  Bus Selector17/1 -> Mux37/1  "<t_0 x>"
  Mux38/1 -> Mux37/4
  Constant59/1 -> Mux38/1
  Constant60/1 -> Mux41/1
  Constant62/1 -> Mux49/2
  Constant68/1 -> Traffic Object21/1
  Bus Selector21/2 -> Mux45/2  "<t_0 y>"
  Mux42/1 -> [Traffic_Info_12]
  Bus Selector20/2 -> Mux42/2  "<t_0 y>"
  Mux49/1 -> Mux42/4
  Traffic Object22/2 -> Bus Selector20/1
  Bus Selector20/1 -> Mux42/1  "<t_0 x>"
  Traffic Object22/1 -> Terminator22/1
  Bus Selector20/3 -> Mux42/3  "<r_zyx z>"
  Constant69/1 -> Mux46/2
  Traffic Object21/2 -> Bus Selector21/1
  Traffic Object21/1 -> Terminator21/1
  Mux45/1 -> [Traffic_Info_05]
  Bus Selector21/3 -> Mux45/3  "<r_zyx z>"
  Constant61/1 -> Traffic Object22/1
  Bus Selector21/1 -> Mux45/1  "<t_0 x>"
  Mux46/1 -> Mux45/4
  Constant71/1 -> Mux46/1
  Constant72/1 -> Mux49/1
  Constant79/1 -> Traffic Object28/1
  Mux52/1 -> [Traffic_Info_27]
  Bus Selector27/1 -> Mux52/1  "<t_0 x>"
  Constant78/1 -> Mux51/2
  Traffic Object28/2 -> Bus Selector27/1
  Constant77/1 -> Mux51/1
  Bus Selector27/3 -> Mux52/3  "<r_zyx z>"
  Constant74/1 -> Mux57/2
  Constant80/1 -> Traffic Object25/1
  Bus Selector25/2 -> Mux53/2  "<t_0 y>"
  Mux50/1 -> [Traffic_Info_13]
  Bus Selector27/2 -> Mux52/2  "<t_0 y>"
  Bus Selector24/2 -> Mux50/2  "<t_0 y>"
  Mux57/1 -> Mux50/4
  Traffic Object26/2 -> Bus Selector24/1
  Bus Selector24/1 -> Mux50/1  "<t_0 x>"
  Traffic Object26/1 -> Terminator26/1
  Bus Selector24/3 -> Mux50/3  "<r_zyx z>"
  Constant81/1 -> Mux54/2
  Traffic Object25/2 -> Bus Selector25/1
  Traffic Object25/1 -> Terminator25/1
  Traffic Object28/1 -> Terminator28/1
  Mux53/1 -> [Traffic_Info_06]
  Bus Selector25/3 -> Mux53/3  "<r_zyx z>"
  Constant73/1 -> Traffic Object26/1
  Bus Selector25/1 -> Mux53/1  "<t_0 x>"
  Mux54/1 -> Mux53/4
  Constant83/1 -> Mux54/1
  Constant84/1 -> Mux57/1
  [Traffic_Info_09] -> Mux9/10  "T09"
  [Traffic_Info_10] -> Mux9/11  "T10"
  [Traffic_Info_11] -> Mux9/12  "T11"
  [Traffic_Info_08] -> Mux9/9  "T08"
  [Traffic_Info_12] -> Mux9/13  "T12"
  [Traffic_Info_13] -> Mux9/14  "T13"
  [Traffic_Info_07] -> Mux9/8  "T07"
  [Traffic_Info_16] -> Mux9/17  "T16"
  [Traffic_Info_17] -> Mux9/18  "T17"
  [Traffic_Info_18] -> Mux9/19  "T18"
  [Traffic_Info_15] -> Mux9/16  "T15"
  [Traffic_Info_19] -> Mux9/20  "T19"
  [Traffic_Info_20] -> Mux9/21  "T20"
  [Traffic_Info_14] -> Mux9/15  "T14"
  [Traffic_Info_23] -> Mux9/24  "T23"
  [Traffic_Info_24] -> Mux9/25  "T24"
  [Traffic_Info_25] -> Mux9/26  "T25"
  [Traffic_Info_22] -> Mux9/23  "T22"
  [Traffic_Info_26] -> Mux9/27  "T26"
  [Traffic_Info_27] -> Mux9/28  "T27"
  [Traffic_Info_21] -> Mux9/22  "T21"

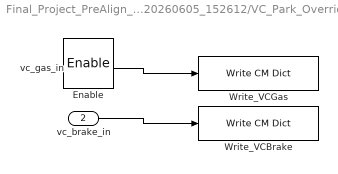
== system Final_Project_PreAlign_20260605_152612/VC_Park_Override ==
  vc_gas_in : Inport
  vc_brake_in : Inport  Port=2
  Enable : EnablePort
  Write_VCBrake : CarMaker4SL/Write CM Dict  xname=VC.Brake  xsync=off
  Write_VCGas : CarMaker4SL/Write CM Dict  xname=VC.Gas  xsync=off
  wires:
  vc_gas_in/1 -> Write_VCGas/1
  vc_brake_in/1 -> Write_VCBrake/1

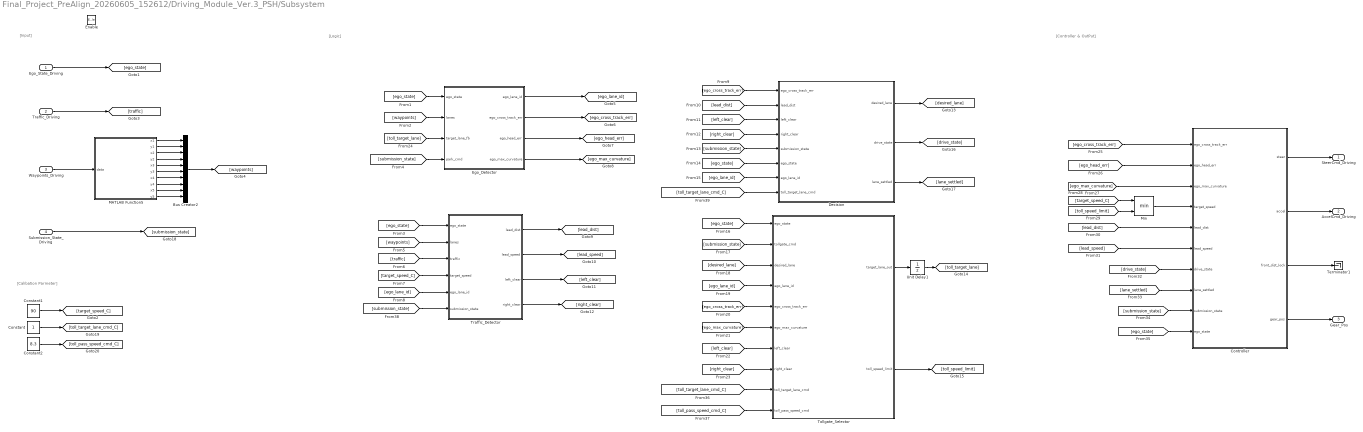
== system Final_Project_PreAlign_20260605_152612/Driving_Module_Ver.3_PSH/Subsystem ==
  note: [Controller & OutPut]
  note: [Logic]
  note: [Input]
  note: [Calibation Parmeter]
  Ego_State_Driving : Inport  OutDataTypeStr=Bus: EgoStateBus
  Traffic_Driving : Inport  Port=2
  Waypoints_Driving : Inport  Port=3
  Submission_State_Driving : Inport  Port=4
  Enable : EnablePort
  Bus Creator2 : BusCreator  Inputs=10  OutDataTypeStr=Bus: ParsedLaneBus
  Constant : Constant
  Constant1 : Constant  Value=90
  Constant2 : Constant  Value=8.3
  Controller : MATLAB Function  TreatAsAtomicUnit=on
  Decision : MATLAB Function  TreatAsAtomicUnit=on
  Ego_Detector : MATLAB Function  TreatAsAtomicUnit=on
  MATLAB Function5 : MATLAB Function  TreatAsAtomicUnit=on
  Min : MinMax  Inputs=2
  Terminator1 : Terminator
  Tollgate_Selector : MATLAB Function  TreatAsAtomicUnit=on
  Traffic_Detector : MATLAB Function  TreatAsAtomicUnit=on
  Unit Delay1 : UnitDelay  InitialCondition=int32(1)  SampleTime=-1  HasFrameUpgradeWarning=on
  SteerCmd_Driving : Outport
  AccelCmd_Driving : Outport  Port=2
  Gear_Pos : Outport  Port=3
  wires:
  [toll_target_lane_cmd_C] -> Decision/8(toll_target_lane_cmd)
  [submission_state] -> Traffic_Detector/6(submission_state)
  [submission_state] -> Decision/5(submission_state)
  [ego_cross_track_err] -> Decision/1(ego_cross_track_err)
  [lead_dist] -> Decision/2(lead_dist)
  [ego_state] -> Decision/6(ego_state)
  Controller/4(gear_pos) -> Gear_Pos/1
  Constant2/1 -> [toll_pass_speed_cmd_C]
  Constant/1 -> [toll_target_lane_cmd_C]
  [toll_pass_speed_cmd_C] -> Tollgate_Selector/10(toll_pass_speed_cmd)
  [toll_target_lane_cmd_C] -> Tollgate_Selector/9(toll_target_lane_cmd)
  Ego_State_Driving/1 -> [ego_state]
  Submission_State_Driving/1 -> [submission_state]
  Tollgate_Selector/1(target_lane_out) -> Unit Delay1/1
  Unit Delay1/1 -> [toll_target_lane]
  Controller/3(front_dist_lock) -> Terminator1/1
  Controller/1(steer) -> SteerCmd_Driving/1
  Controller/2(accel) -> AccelCmd_Driving/1
  [ego_state] -> Controller/10(ego_state)
  [submission_state] -> Controller/9(submission_state)
  [lane_settled] -> Controller/8(lane_settled)
  [drive_state] -> Controller/7(drive_state)
  [lead_speed] -> Controller/6(lead_speed)
  [lead_dist] -> Controller/5(lead_dist)
  [toll_speed_limit] -> Min/2
  [target_speed_C] -> Min/1
  Min/1 -> Controller/4(target_speed)
  [ego_max_curvature] -> Controller/3(ego_max_curvature)
  [ego_head_err] -> Controller/2(ego_head_err)
  [ego_cross_track_err] -> Controller/1(ego_cross_track_err)
  Decision/2(drive_state) -> [drive_state]
  Decision/3(lane_settled) -> [lane_settled]
  [toll_target_lane] -> Ego_Detector/3(target_lane_fb)
  Tollgate_Selector/2(toll_speed_limit) -> [toll_speed_limit]
  [right_clear] -> Tollgate_Selector/8(right_clear)
  [left_clear] -> Tollgate_Selector/7(left_clear)
  [ego_max_curvature] -> Tollgate_Selector/6(ego_max_curvature)
  [ego_cross_track_err] -> Tollgate_Selector/5(ego_cross_track_err)
  [ego_lane_id] -> Tollgate_Selector/4(ego_lane_id)
  [desired_lane] -> Tollgate_Selector/3(desired_lane)
  Decision/1(desired_lane) -> [desired_lane]
  [submission_state] -> Tollgate_Selector/2(tollgate_cmd)
  [ego_state] -> Tollgate_Selector/1(ego_state)
  [ego_lane_id] -> Decision/7(ego_lane_id)
  [right_clear] -> Decision/4(right_clear)
  [left_clear] -> Decision/3(left_clear)
  Traffic_Detector/4(right_clear) -> [right_clear]
  Traffic_Detector/3(left_clear) -> [left_clear]
  Traffic_Detector/2(lead_speed) -> [lead_speed]
  Traffic_Detector/1(lead_dist) -> [lead_dist]
  [ego_lane_id] -> Traffic_Detector/5(ego_lane_id)
  [target_speed_C] -> Traffic_Detector/4(target_speed)
  [traffic] -> Traffic_Detector/3(traffic)
  [waypoints] -> Traffic_Detector/2(lanes)
  [ego_state] -> Traffic_Detector/1(ego_state)
  Ego_Detector/2(ego_cross_track_err) -> [ego_cross_track_err]
  Ego_Detector/3(ego_head_err) -> [ego_head_err]
  Ego_Detector/4(ego_max_curvature) -> [ego_max_curvature]
  Ego_Detector/1(ego_lane_id) -> [ego_lane_id]
  [waypoints] -> Ego_Detector/2(lanes)
  [ego_state] -> Ego_Detector/1(ego_state)
  [submission_state] -> Ego_Detector/4(park_cmd)
  Bus Creator2/1 -> [waypoints]
  MATLAB Function5/10(y5) -> Bus Creator2/10
  MATLAB Function5/9(x5) -> Bus Creator2/9
  MATLAB Function5/8(y4) -> Bus Creator2/8
  MATLAB Function5/7(x4) -> Bus Creator2/7
  MATLAB Function5/6(y3) -> Bus Creator2/6
  MATLAB Function5/5(x3) -> Bus Creator2/5
  MATLAB Function5/4(y2) -> Bus Creator2/4
  MATLAB Function5/3(x2) -> Bus Creator2/3
  MATLAB Function5/2(y1) -> Bus Creator2/2
  MATLAB Function5/1(x1) -> Bus Creator2/1
  Waypoints_Driving/1 -> MATLAB Function5/1(data)
  Traffic_Driving/1 -> [traffic]
  Constant1/1 -> [target_speed_C]

== matlab function Final_Project_PreAlign_20260605_152612/Driving_Module_Ver.3_PSH/Subsystem/MATLAB Function5 ==
  data: data input; x1 output; y1 output; x2 output; y2 output; x3 output; y3 output; x4 output; y4 output; x5 output; y5 output
function [x1,y1,x2,y2,x3,y3,x4,y4,x5,y5] = parse_lane(data)
%#codegen
    % waypoints_classified_line.xlsx 기준
    % column 1: id
    % column 2: global_x
    % column 3: global_y
    % column 4: line

    N1 = 283;
    N2 = 275;
    N3 = 266;
    N4 = 34;
    N5 = 19;

    x1 = zeros(N1, 1);
    y1 = zeros(N1, 1);

    x2 = zeros(N2, 1);
    y2 = zeros(N2, 1);

    x3 = zeros(N3, 1);
    y3 = zeros(N3, 1);

    x4 = zeros(N4, 1);
    y4 = zeros(N4, 1);

    x5 = zeros(N5, 1);
    y5 = zeros(N5, 1);

    i1 = int32(0);
    i2 = int32(0);
    i3 = int32(0);
    i4 = int32(0);
    i5 = int32(0);

    N = int32(size(data, 1));

    for k = 1:N
        lk = data(k, 4);
        xk = data(k, 2);
        yk = data(k, 3);

        if lk == 1
            if i1 < int32(N1)
                i1 = i1 + int32(1);
                x1(i1) = xk;
                y1(i1) = yk;
            end

        elseif lk == 2
            if i2 < int32(N2)
                i2 = i2 + int32(1);
                x2(i2) = xk;
                y2(i2) = yk;
            end

        elseif lk == 3
            if i3 < int32(N3)
                i3 = i3 + int32(1);
                x3(i3) = xk;
                y3(i3) = yk;
            end

        elseif lk == 4
            if i4 < int32(N4)
                i4 = i4 + int32(1);
                x4(i4) = xk;
                y4(i4) = yk;
            end

        elseif lk == 5
            if i5 < int32(N5)
                i5 = i5 + int32(1);
                x5(i5) = xk;
                y5(i5) = yk;
            end
        end
    end
end

== matlab function Final_Project_PreAlign_20260605_152612/Driving_Module_Ver.3_PSH/Subsystem/Ego_Detector ==
  data: ego_state input; ego_lane_id output; lanes input; target_lane_fb input; ego_cross_track_err output; ego_head_err output; ego_max_curvature output; park_cmd input
function [ego_lane_id, ego_cross_track_err, ego_head_err, ego_max_curvature] = Ego_Detector(ego_state, lanes, target_lane_fb, park_cmd)
%#codegen

    % ============================================================
    % 1. EgoStateBus unpack
    % ============================================================
    ego_x   = ego_state.Car_Fr1_tx;
    ego_y   = ego_state.Car_Fr1_ty;
    ego_yaw = ego_state.Car_Fr1_rz;

    % ============================================================
    % 2. ParsedLaneBus unpack - 5차선
    % ============================================================
    x1 = lanes.x1;  y1 = lanes.y1;
    x2 = lanes.x2;  y2 = lanes.y2;
    x3 = lanes.x3;  y3 = lanes.y3;
    x4 = lanes.x4;  y4 = lanes.y4;
    x5 = lanes.x5;  y5 = lanes.y5;

    % lane5 좌측 보정
    L5_OFFSET = 1.0;
    x5 = x5 + L5_OFFSET;

    % ============================================================
    % 3. 현재 ego가 가장 가까운 차선 판단
    % ============================================================
    d1 = nearest_d2(x1, y1, ego_x, ego_y);
    d2 = nearest_d2(x2, y2, ego_x, ego_y);
    d3 = nearest_d2(x3, y3, ego_x, ego_y);
    d4 = nearest_d2(x4, y4, ego_x, ego_y);
    d5 = nearest_d2(x5, y5, ego_x, ego_y);

    ego_lane_id = int32(1);
    dmin = d1;

    if d2 < dmin
        dmin = d2;
        ego_lane_id = int32(2);
    end

    if d3 < dmin
        dmin = d3;
        ego_lane_id = int32(3);
    end

    if d4 < dmin
        dmin = d4;
        ego_lane_id = int32(4);
    end

    if d5 < dmin
        ego_lane_id = int32(5);
    end

    % ============================================================
    % 4. target_lane 보호
    % ============================================================
    target_lane = int32(target_lane_fb);

    if target_lane < int32(1)
        target_lane = int32(1);
    elseif target_lane > int32(5)
        target_lane = int32(5);
    end

    % ============================================================
    % 5. 주차 진입 구간에서는 preview step 축소
    % ============================================================
    if park_cmd == int32(1) && ...
       (target_lane == int32(4) || target_lane == int32(5))
        LOOK_STEP = int32(2);
    else
        LOOK_STEP = int32(5);
    end

    % ============================================================
    % 6. target lane 기준 오차 / 곡률 계산
    % ============================================================
    if target_lane == int32(1)

        [ego_cross_track_err, ego_head_err, ego_max_curvature] = process_lane_closed( ...
            x1, y1, ego_x, ego_y, ego_yaw, LOOK_STEP);

    elseif target_lane == int32(2)

        [ego_cross_track_err, ego_head_err, ego_max_curvature] = process_lane_closed( ...
            x2, y2, ego_x, ego_y, ego_yaw, LOOK_STEP);

    elseif target_lane == int32(3)

        [ego_cross_track_err, ego_head_err, ego_max_curvature] = process_lane_closed( ...
            x3, y3, ego_x, ego_y, ego_yaw, LOOK_STEP);

    elseif target_lane == int32(4)

        [ego_cross_track_err, ego_head_err, ego_max_curvature] = process_lane_open( ...
            x4, y4, ego_x, ego_y, ego_yaw, LOOK_STEP);

    else

        [ego_cross_track_err, ego_head_err, ego_max_curvature] = process_lane_open( ...
            x5, y5, ego_x, ego_y, ego_yaw, LOOK_STEP);

    end

    % ============================================================
    % 7. [추가] 주차 진입차선(4/5)에서 우측차선에 딱붙어 진입
    %    controller가 cross_track_err->0 추종하므로, err에 offset을 더하면
    %    ego가 차선중심에서 그 반대방향으로 hold됨 (= 우측 hugging).
    %    부호/크기는 테스트로 확정.
    % ============================================================
    HUG_RIGHT_OFFSET = 1.2;   % [튜닝] 우측 오프셋[m]
    if park_cmd == int32(1) && (target_lane == int32(4) || target_lane == int32(5))
        ego_cross_track_err = ego_cross_track_err + HUG_RIGHT_OFFSET;
    end

end


function d2 = nearest_d2(xa, ya, ex, ey)
%#codegen

    d2 = 1e12;
    N  = int32(numel(xa));

    for i = 1:N
        dxk = xa(i) - ex;
        dyk = ya(i) - ey;
        v   = dxk*dxk + dyk*dyk;

        if v < d2
            d2 = v;
        end
    end

end


function [ego_cross_track_err, ego_head_err, ego_max_curvature] = process_lane_open(xa, ya, ex, ey, eyaw, LOOK_STEP)
%#codegen

    N = int32(numel(xa));

    best_i  = int32(1);
    best_d2 = 1e12;

    for i = 1:N
        dxk = xa(i) - ex;
        dyk = ya(i) - ey;
        v   = dxk*dxk + dyk*dyk;

        if v < best_d2
            best_d2 = v;
            best_i  = i;
        end
    end

    look_i = best_i + LOOK_STEP;

    if look_i > N
        look_i = N;
    end

    if look_i > best_i

        path_yaw = atan2( ...
            ya(look_i) - ya(best_i), ...
            xa(look_i) - xa(best_i));

    elseif best_i > int32(1)

        path_yaw = atan2( ...
            ya(best_i) - ya(best_i - int32(1)), ...
            xa(best_i) - xa(best_i - int32(1)));

    else

        path_yaw = eyaw;

    end

    dxr = ex - xa(best_i);
    dyr = ey - ya(best_i);

    ego_cross_track_err = -sin(path_yaw) * dxr + cos(path_yaw) * dyr;

    ego_head_err = wrap_pi(path_yaw - eyaw);

    ego_max_curvature = 0.0;
    STEP = int32(5);

    for kk = 0:4
        base_i = best_i + int32(kk) * STEP;

        i1 = base_i;
        i2 = base_i + STEP;
        i3 = base_i + int32(2) * STEP;

        if i1 > N
            i1 = N;
        end

        if i2 > N
            i2 = N;
        end

        if i3 > N
            i3 = N;
        end

        if i1 < i2 && i2 < i3

            yaw1 = atan2( ...
                ya(i2) - ya(i1), ...
                xa(i2) - xa(i1));

            yaw2 = atan2( ...
                ya(i3) - ya(i2), ...
                xa(i3) - xa(i2));

            dyaw = wrap_pi(yaw2 - yaw1);

            ds = sqrt( ...
                (xa(i3) - xa(i1))^2 + ...
                (ya(i3) - ya(i1))^2);

            if ds > 0.1
                kappa = abs(dyaw) / ds;

                if kappa > ego_max_curvature
                    ego_max_curvature = kappa;
                end
            end
        end
    end

end


function [ego_cross_track_err, ego_head_err, ego_max_curvature] = process_lane_closed(xa, ya, ex, ey, eyaw, LOOK_STEP)
%#codegen

    N = int32(numel(xa));

    best_i  = int32(1);
    best_d2 = 1e12;

    for i = 1:N
        dxk = xa(i) - ex;
        dyk = ya(i) - ey;
        v   = dxk*dxk + dyk*dyk;

        if v < best_d2
            best_d2 = v;
            best_i  = i;
        end
    end

    look_i = wrap_idx(best_i + LOOK_STEP, N);

    path_yaw = atan2( ...
        ya(look_i) - ya(best_i), ...
        xa(look_i) - xa(best_i));

    dxr = ex - xa(best_i);
    dyr = ey - ya(best_i);

    ego_cross_track_err = -sin(path_yaw) * dxr + cos(path_yaw) * dyr;

    ego_head_err = wrap_pi(path_yaw - eyaw);

    ego_max_curvature = 0.0;
    STEP = int32(5);

    for kk = 0:4
        base_i = wrap_idx(best_i + int32(kk) * STEP, N);

        i1 = base_i;
        i2 = wrap_idx(base_i + STEP, N);
        i3 = wrap_idx(base_i + int32(2) * STEP, N);

        yaw1 = atan2( ...
            ya(i2) - ya(i1), ...
            xa(i2) - xa(i1));

        yaw2 = atan2( ...
            ya(i3) - ya(i2), ...
            xa(i3) - xa(i2));

        dyaw = wrap_pi(yaw2 - yaw1);

        ds = sqrt( ...
            (xa(i3) - xa(i1))^2 + ...
            (ya(i3) - ya(i1))^2);

        if ds > 0.1
            kappa = abs(dyaw) / ds;

            if kappa > ego_max_curvature
                ego_max_curvature = kappa;
            end
        end
    end

end


function idx = wrap_idx(idx_in, N)
%#codegen
    idx = idx_in;

    while idx > N
        idx = idx - N;
    end

    while idx < int32(1)
        idx = idx + N;
    end

end


function a = wrap_pi(a)
%#codegen

    while a > pi
        a = a - 2.0*pi;
    end

    while a < -pi
        a = a + 2.0*pi;
    end

end
